simulink model "esempio1_farrell"  (R2025b)
settings: Solver=ode45  StartTime=0.0  StopTime=100  RelTol=1e-3  EnableMultiTasking=on
values from neighbouring files (symbols this model uses):
  C = 40    [Lab7.m]
  c1 = -1    [Lab7.m]
  c2 = -0.5    [Lab7.m]
  c3 = 0    [Lab7.m]
  c4 = 0.5    [Lab7.m]
  c5 = 1    [Lab7.m]
  G = 1/20    (= 0.05)    [Lab7.m]
  gamma_f = 100    [Lab7.m]
  gamma_g = 10    [Lab7.m]
  s1 = s_val    (= 0.5)    [Lab7.m]
  s2 = s_val    (= 0.5)    [Lab7.m]
  s3 = s_val    (= 0.5)    [Lab7.m]
  s4 = s_val    (= 0.5)    [Lab7.m]
  s5 = s_val    (= 0.5)    [Lab7.m]
  Teta_f0 = zeros(5, 1)    [Lab7.m]
  Teta_g0 = ones(5, 1)*0.5    [Lab7.m]
libraries: simulink x1
settings Model: Creator=C.Perri  LastModifiedBy=Steph
settings SolverCC: AlgebraicLoopSolver=TrustRegion
settings DataIOCC: LimitDataPoints=on  SaveFormat=Array  SignalLoggingSaveFormat=ModelDataLogs  ReturnWorkspaceOutputs=off
settings OptimizationCC: InitFltsAndDblsToZero=on  LifeSpan=inf
settings DebuggingCC: SaveWithParameterizedLinksMsg=none  UnderspecifiedInitializationDetection=Classic  MergeDetectMultiDrivingBlocksExec=none  SignalResolutionControl=TryResolveAllWithWarning  SolverPrmCheckMsg=warning  MultiTaskDSMMsg=warning  MultiTaskCondExecSysMsg=none  FcnCallInpInsideContextMsg=warning  UnconnectedInputMsg=warning  UnconnectedOutputMsg=warning  UnconnectedLineMsg=warning  SFUnexpectedBacktrackingDiag=warning  SFNoUnconditionalDefaultTransitionDiag=warning  SFExecutionAtInitializationDiag=none  ArithmeticOperatorsInVariantConditions=warning
settings HardwareCC: ProdBitPerPointer=32.0  ProdBitPerSizeT=32.0  ProdBitPerPtrDiffT=32.0  ProdLargestAtomicFloat=None  ProdIntDivRoundTo=Undefined  ProdEndianess=Unspecified  ProdWordSize=32.0  ProdHWDeviceType=32-bit Generic
settings ModelReferenceCC: EnableRefExpFcnMdlSchedulingChecks=on  PropagateSignalLabelsOutOfModel=off
settings RTWCC: GPUComputeCapability=3.5
settings CodeAppCC: StateflowObjectComments=on
settings GRTTargetCC: TargetFcnLib=ansi_tfl_tmw.mat  TargetLangStandard=C89/C90 (ANSI)  CombineOutputUpdateFcns=off  GRTInterface=on
settings ConfigComp: CovMetricSettings=dw  CovSaveCumulativeToWorkspaceVar=on  CovSaveSingleToWorkspaceVar=on

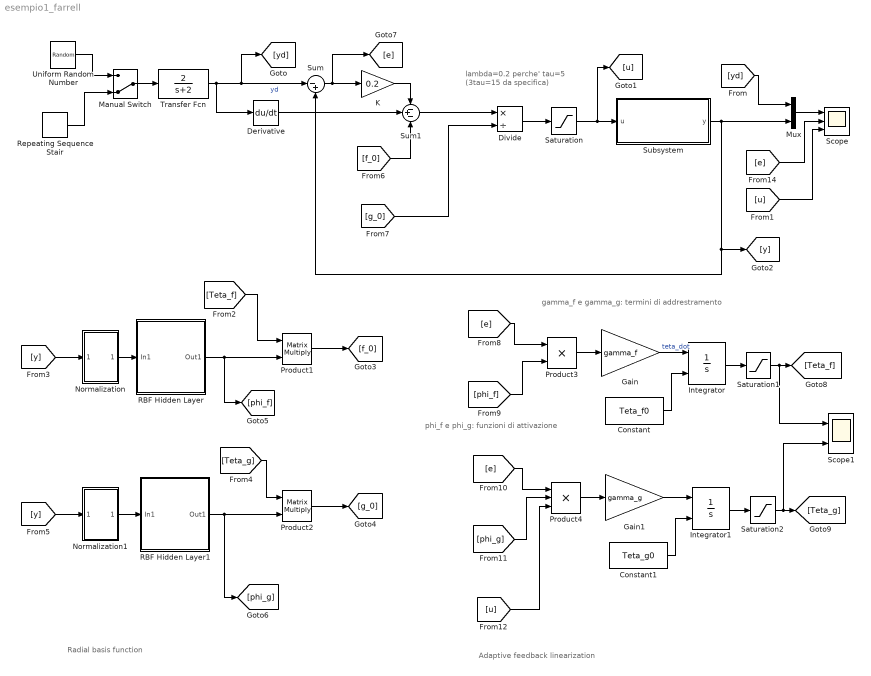
== system esempio1_farrell ==
  note: phi_f e phi_g: funzioni di attivazione
  note: gamma_f e gamma_g: termini di addrestramento
  note: Adaptive feedback linearization
  note: lambda=0.2 perche'
      | tau=5 (3tau=15 da specifica)
  note: Radial basis function
  Constant : Constant  Value=Teta_f0
  Constant1 : Constant  Value=Teta_g0
  Derivative : Derivative
  Divide : Product  Inputs=*/
  Gain : Gain  Gain=gamma_f
  Gain1 : Gain  Gain=gamma_g
  Integrator : Integrator  InitialConditionSource=external
  Integrator1 : Integrator  InitialConditionSource=external
  K : Gain  Gain=0.2
  Manual Switch : ManualSwitch  CurrentSetting=0
  Mux : Mux  Inputs=2
  Normalization : Subsystem
  Normalization1 : Subsystem
  Product1 : Product  Multiplication=Matrix(*)  RndMeth=Zero
  Product2 : Product  Multiplication=Matrix(*)  RndMeth=Zero
  Product3 : Product  RndMeth=Zero
  Product4 : Product  Inputs=3  RndMeth=Zero
  RBF Hidden Layer : Subsystem
  RBF Hidden Layer1 : Subsystem
  Repeating Sequence Stair : simulink/Sources/Repeating Sequence Stair  OutValues=[20 60].'  tsamp=10  OutMin=[]  OutMax=[]  OutDataTypeStr=float('double')  OutputDataTypeScalingMode=Specify via dialog  OutDataType=float('double')  ConRadixGroup=Best Precision: Vector-wise  OutScaling=2^-12
  Saturation : Saturate  UpperLimit=10  LowerLimit=-10
  Saturation1 : Saturate  UpperLimit=30  LowerLimit=-30
  Saturation2 : Saturate  UpperLimit=15  LowerLimit=0.1
  Scope : Scope  NumInputPorts=3
      settings: ActiveDisplayYMinimum=-7.5632083900972216  ActiveDisplayYMaximum=68.068875510875017
  Scope1 : Scope  NumInputPorts=2
      settings: TimeSpan=100  ActiveDisplayYMinimum=-71.38391  ActiveDisplayYMaximum=42.5905
  Subsystem : Subsystem
  Sum : Sum  Inputs=|-+
  Sum1 : Sum  Inputs=-+-
  Transfer Fcn : TransferFcn  Numerator=[2]  Denominator=[1 2]
  Uniform Random Number : UniformRandomNumber  Minimum=20  Maximum=60  SampleTime=3
  wires:
  Subsystem/1(y) -> Mux/2, Sum/2, [y]
  Transfer Fcn/1 -> Derivative/1, Sum/1, [yd]  "yd"
  Sum/1 -> K/1, [e]
  K/1 -> Sum1/1
  Derivative/1 -> Sum1/2
  [yd] -> Mux/1
  Mux/1 -> Scope/1
  Sum1/1 -> Divide/1
  Divide/1 -> Saturation/1
  Manual Switch/1 -> Transfer Fcn/1
  Uniform Random Number/1 -> Manual Switch/1
  Repeating Sequence Stair/1 -> Manual Switch/2
  Saturation/1 -> Subsystem/1(u), [u]
  [f_0] -> Sum1/3
  RBF Hidden Layer/1(Out1) -> Product1/2, [phi_f]
  Product1/1 -> [f_0]
  [y] -> Normalization/1(In1)
  Normalization/1(Out1) -> RBF Hidden Layer/1(In1)
  RBF Hidden Layer1/1(Out1) -> Product2/2, [phi_g]
  Product2/1 -> [g_0]
  [y] -> Normalization1/1(In1)
  Normalization1/1(Out1) -> RBF Hidden Layer1/1(In1)
  [Teta_f] -> Product1/1
  [Teta_g] -> Product2/1
  Product3/1 -> Gain/1
  [e] -> Product3/1
  [phi_f] -> Product3/2
  Gain/1 -> Integrator/1  "teta_dot"
  Integrator/1 -> Saturation1/1
  Saturation1/1 -> [Teta_f], Scope1/1
  Constant/1 -> Integrator/2
  Product4/1 -> Gain1/1
  [e] -> Product4/1
  [phi_g] -> Product4/2
  Gain1/1 -> Integrator1/1
  Integrator1/1 -> Saturation2/1
  Saturation2/1 -> [Teta_g], Scope1/2
  Constant1/1 -> Integrator1/2
  [u] -> Scope/3
  [e] -> Scope/2
  [g_0] -> Divide/2
  [u] -> Product4/3

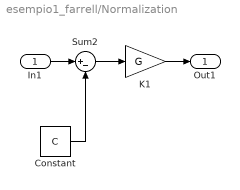
== system esempio1_farrell/Normalization ==
  In1 : Inport
  Constant : Constant  Value=C
  K1 : Gain  Gain=G
  Sum2 : Sum  Inputs=|+-
  Out1 : Outport
  wires:
  In1/1 -> Sum2/1
  K1/1 -> Out1/1
  Constant/1 -> Sum2/2
  Sum2/1 -> K1/1

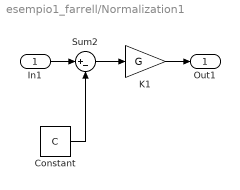
== system esempio1_farrell/Normalization1 ==
  In1 : Inport
  Constant : Constant  Value=C
  K1 : Gain  Gain=G
  Sum2 : Sum  Inputs=|+-
  Out1 : Outport
  wires:
  Sum2/1 -> K1/1
  Constant/1 -> Sum2/2
  K1/1 -> Out1/1
  In1/1 -> Sum2/1

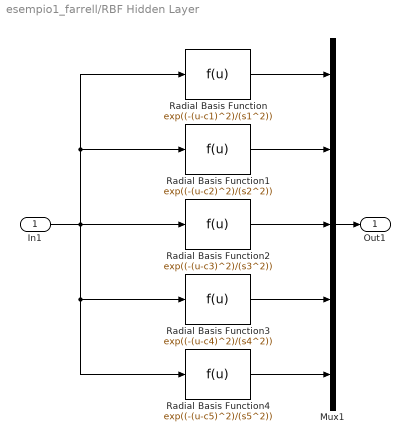
== system esempio1_farrell/RBF Hidden Layer ==
  In1 : Inport
  Mux1 : Mux  Inputs=5
  Radial Basis Function : Fcn  Expr=exp((-(u-c1)^2)/(s1^2))
  Radial Basis Function1 : Fcn  Expr=exp((-(u-c2)^2)/(s2^2))
  Radial Basis Function2 : Fcn  Expr=exp((-(u-c3)^2)/(s3^2))
  Radial Basis Function3 : Fcn  Expr=exp((-(u-c4)^2)/(s4^2))
  Radial Basis Function4 : Fcn  Expr=exp((-(u-c5)^2)/(s5^2))
  Out1 : Outport
  wires:
  Mux1/1 -> Out1/1
  In1/1 -> Radial Basis Function4/1, Radial Basis Function3/1, Radial Basis Function/1, Radial Basis Function1/1, Radial Basis Function2/1
  Radial Basis Function4/1 -> Mux1/5
  Radial Basis Function3/1 -> Mux1/4
  Radial Basis Function2/1 -> Mux1/3
  Radial Basis Function1/1 -> Mux1/2
  Radial Basis Function/1 -> Mux1/1

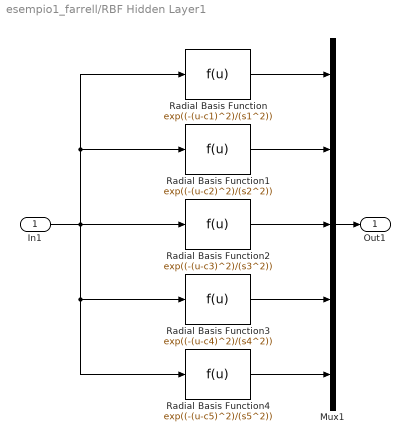
== system esempio1_farrell/RBF Hidden Layer1 ==
  In1 : Inport
  Mux1 : Mux  Inputs=5
  Radial Basis Function : Fcn  Expr=exp((-(u-c1)^2)/(s1^2))
  Radial Basis Function1 : Fcn  Expr=exp((-(u-c2)^2)/(s2^2))
  Radial Basis Function2 : Fcn  Expr=exp((-(u-c3)^2)/(s3^2))
  Radial Basis Function3 : Fcn  Expr=exp((-(u-c4)^2)/(s4^2))
  Radial Basis Function4 : Fcn  Expr=exp((-(u-c5)^2)/(s5^2))
  Out1 : Outport
  wires:
  Radial Basis Function/1 -> Mux1/1
  Radial Basis Function1/1 -> Mux1/2
  Radial Basis Function2/1 -> Mux1/3
  Radial Basis Function3/1 -> Mux1/4
  Radial Basis Function4/1 -> Mux1/5
  In1/1 -> Radial Basis Function2/1, Radial Basis Function1/1, Radial Basis Function/1, Radial Basis Function3/1, Radial Basis Function4/1
  Mux1/1 -> Out1/1

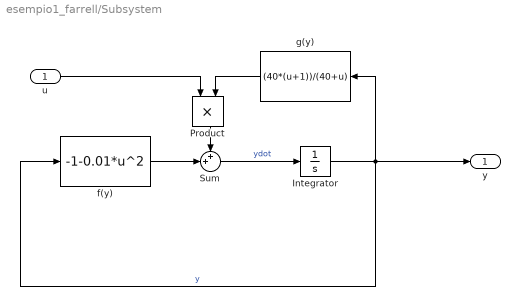
== system esempio1_farrell/Subsystem ==
  u : Inport
  Integrator : Integrator
  Product : Product  RndMeth=Zero
  Sum : Sum  Inputs=++|
  f(y) : Fcn  Expr=-1-0.01*u^2
  g(y) : Fcn  Expr=(40*(u+1))/(40+u)
  y : Outport
  wires:
  Sum/1 -> Integrator/1  "ydot"
  f(y)/1 -> Sum/2
  Product/1 -> Sum/1
  g(y)/1 -> Product/2
  u/1 -> Product/1
  Integrator/1 -> y/1, g(y)/1, f(y)/1  "y"
